simulink subsystem "Environment_Model"  (R2024b)
settings: Solver=VariableStepAuto  StartTime=0.0  StopTime=10.0  RelTol=1e-3
values from neighbouring files (symbols this model uses):
  r = 0    [Barrowman_Equations.m]    (also in barrowaman.mat = 1.08571428571)
  v_w_avg = 2    [Barrowman_Equations.m]    (also in barrowaman.mat)
  wind_dir = 0    [Barrowman_Equations.m]    (also in barrowaman.mat)
undefined symbols (not defined in the file or in its folder): Earth, F, Light, MIL, WGS84
libraries: aerolibwind2 x2, aerolibatmos2 x1, aerolibtransform2 x1
settings Model: Creator=joedo  LastModifiedBy=trist

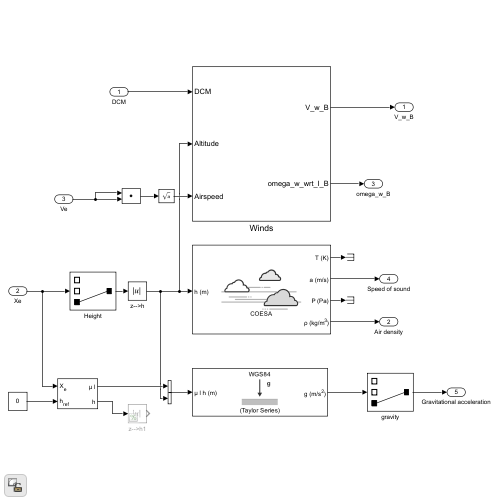
[thumbnail: Simulink's stored preview of the top-level diagram]
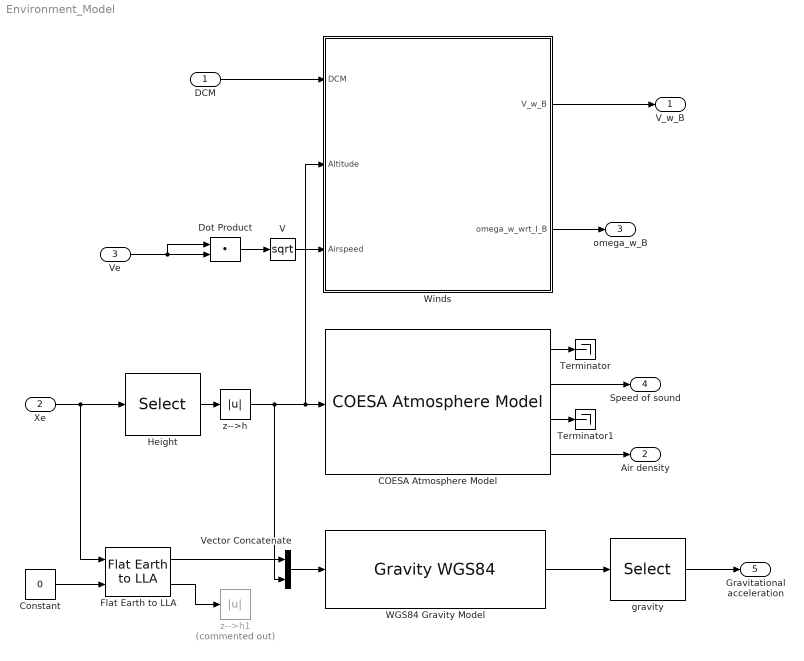
== system Environment_Model ==
  DCM : Inport
  Xe : Inport  Port=2
  Ve : Inport  Port=3
  COESA Atmosphere Model : aerolibatmos2/COESA Atmosphere Model  units=Metric (MKS)  spec=1976 COESA-extended U.S. Standard Atmosphere  model=Profile  profile_var=High temperature  profile_percent=10%  profile_alt=5 km (16404 ft)  envelope_var=High temperature  envelope_percent=1%  action=None
  Constant : Constant  Value=0
  Dot Product : DotProduct  SaturateOnIntegerOverflow=on  InputSameDT=off  OutDataTypeStr=Inherit: Inherit via internal rule
  Flat Earth to LLA : aerolibtransform2/Flat Earth to LLA  units=Metric (MKS)  ptype=Earth (WGS84)  F=1/298.257223563  R=6378137  refPosPort=off  LL0=[43.4643 -80.5204]  psi=0
  Height : Selector  InputPortWidth=3  IndexOptions=Index vector (dialog)  Indices=[3]  OutputSizes=1
  Terminator : Terminator
  Terminator1 : Terminator
  V : Math  Operator=sqrt  SignedPower=on
  Vector Concatenate : Concatenate
  "WGS84 Gravity Model  " : GravityWGS84  action=Error
  Winds : Subsystem
  gravity : Selector  InputPortWidth=3  IndexOptions=Index vector (dialog)  Indices=[3]  OutputSizes=1
  z-->h : Abs
  z-->h1 : Abs  Commented=on
  V_w_B : Outport  VectorParamsAs1DForOutWhenUnconnected=off
  Air density : Outport  Port=2  VectorParamsAs1DForOutWhenUnconnected=off
  omega_w_B : Outport  Port=3  VectorParamsAs1DForOutWhenUnconnected=off
  Speed of sound : Outport  Port=4  VectorParamsAs1DForOutWhenUnconnected=off
  Gravitational acceleration : Outport  Port=5
  wires:
  z-->h/1 -> COESA Atmosphere Model/1, Winds/2(Altitude), Vector Concatenate/2
  Winds/2(omega_w_wrt_I_B) -> omega_w_B/1
  DCM/1 -> Winds/1(DCM)
  Ve/1 -> Dot Product/2, Dot Product/1
  Dot Product/1 -> V/1
  V/1 -> Winds/3(Airspeed)
  COESA Atmosphere Model/2 -> Speed of sound/1
  COESA Atmosphere Model/3 -> Terminator1/1
  COESA Atmosphere Model/1 -> Terminator/1
  COESA Atmosphere Model/4 -> Air density/1
  Height/1 -> z-->h/1
  Xe/1 -> Height/1, Flat Earth to LLA/1
  "WGS84 Gravity Model  "/1 -> gravity/1
  Constant/1 -> Flat Earth to LLA/2
  Flat Earth to LLA/1 -> Vector Concatenate/1
  Flat Earth to LLA/2 -> z-->h1/1
  Vector Concatenate/1 -> "WGS84 Gravity Model  "/1
  gravity/1 -> Gravitational acceleration/1
  Winds/1(V_w_B) -> V_w_B/1

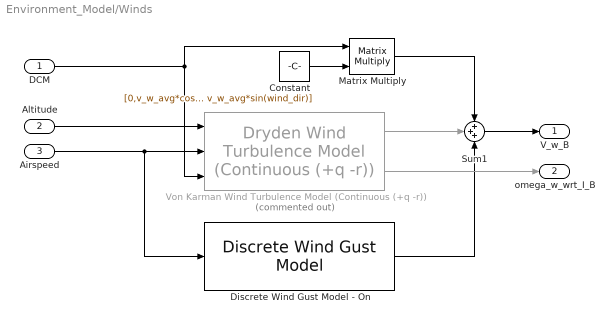
== system Environment_Model/Winds ==
  DCM : Inport
  Altitude : Inport  Port=2
  Airspeed : Inport  Port=3
  Constant : Constant  Value=[0,v_w_avg*cos(wind_dir), v_w_avg*sin(wind_dir)]
  Discrete Wind Gust Model - On : aerolibwind2/Discrete Wind Gust Model  units=Metric (MKS)  Gx=on  Gy=on  Gz=on  t_0=20  d_m=[120 120 80]  v_m=[3.5 3.0 3.0]
  Matrix Multiply : Product  Multiplication=Matrix(*)
  Sum1 : Sum  Inputs=+++  InputSameDT=on  SaturateOnIntegerOverflow=on  OutDataTypeStr=Inherit: Same as first input
  Von Karman Wind Turbulence Model (Continuous (+q -r)) : aerolibwind2/Dryden Wind Turbulence Model  (Continuous (+q -r))  Commented=on  units=Metric (MKS)  spec=MIL-F-8785C  model=Discrete Dryden (+q -r)  W20=v_w_avg  Wdeg=wind_dir  TurbProb=10^-2 - Light  L_high=762  Wingspan=0.5  ts=1  Seed=[23341 23342 23343 23344]  T_on=on
  V_w_B : Outport  VectorParamsAs1DForOutWhenUnconnected=off
  omega_w_wrt_I_B : Outport  Port=2  VectorParamsAs1DForOutWhenUnconnected=off
  wires:
  Matrix Multiply/1 -> Sum1/1
  Von Karman Wind Turbulence Model (Continuous (+q -r))/1 -> Sum1/2
  Altitude/1 -> Von Karman Wind Turbulence Model (Continuous (+q -r))/1
  Sum1/1 -> V_w_B/1
  Airspeed/1 -> Discrete Wind Gust Model - On/1, Von Karman Wind Turbulence Model (Continuous (+q -r))/2
  DCM/1 -> Von Karman Wind Turbulence Model (Continuous (+q -r))/3, Matrix Multiply/1
  Discrete Wind Gust Model - On/1 -> Sum1/3
  Constant/1 -> Matrix Multiply/2
  Von Karman Wind Turbulence Model (Continuous (+q -r))/2 -> omega_w_wrt_I_B/1
